simulink model "Fuzzy_and_EKF"  (R2021b)
settings: Solver=ode4  StartTime=0.0  StopTime=25  FixedStep=1e-2  RelTol=1e-3
values from neighbouring files (symbols this model uses):
  n = length(out.tout)    [Plot_dati.m]    (also in sensors_model.m = 2)
undefined symbols (not defined in the file or in its folder): measure
libraries: fuzblock x1
settings Model: Creator=francescoiotti  LastModifiedBy=francescoiotti
settings ModelReferenceCC: ModelReferenceMinAlgLoopOccurrences=on

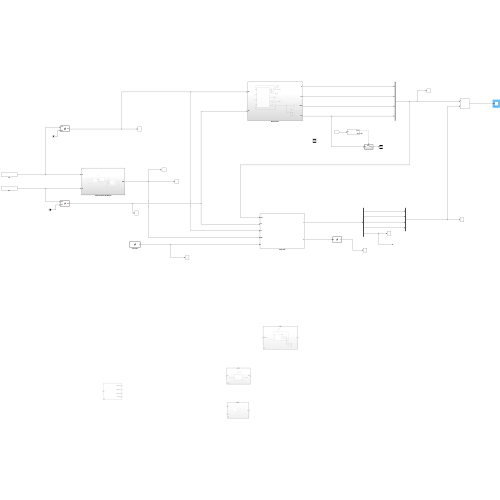
[thumbnail: Simulink's stored preview of the top-level diagram]
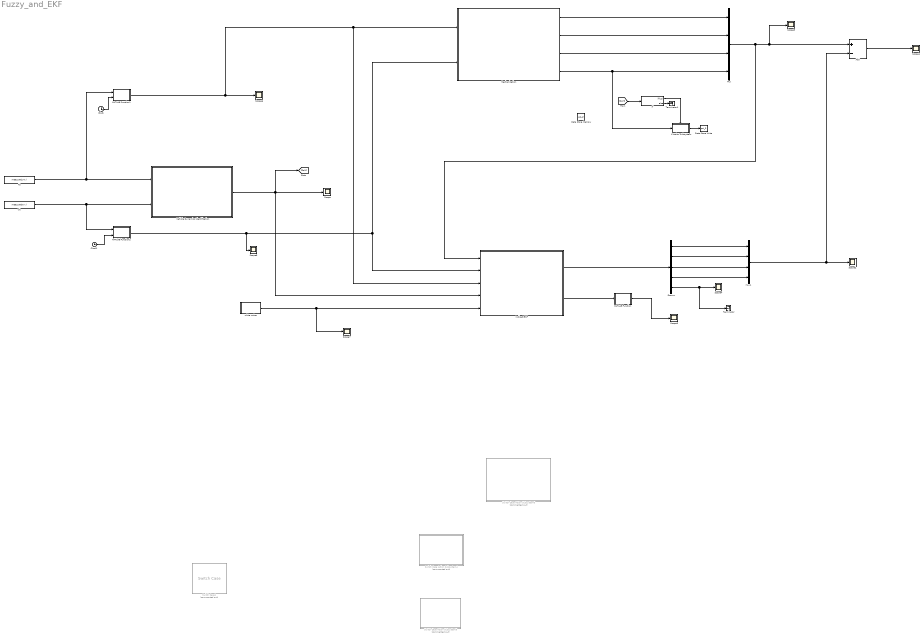
== system Fuzzy_and_EKF ==
  Ab : Constant  Value=measure(2:4,:)
  Add : Sum  Inputs=+-
  Clock : Clock
  Clock1 : Clock
  Data Store Memory : DataStoreMemory  DataStoreName=psi_P  ReadBeforeWriteMsg=warning  WriteAfterWriteMsg=warning  WriteAfterReadMsg=warning  ShowAdditionalParam=off
  Data Store Write : DataStoreWrite  DataStoreName=psi_P  IndexOptions=Index vector (dialog)  Indices=1  OutputSizes=1
  Demux : Demux  Outputs=5
  If : If  IfExpression=u1
  If Action Subsystem : Subsystem  TreatAsAtomicUnit=on
  Indirect EKF : Subsystem
  MATLAB Function : MATLAB Function  TreatAsAtomicUnit=on
  MATLAB Function1 : MATLAB Function  TreatAsAtomicUnit=on
  MATLAB Function2 : MATLAB Function  TreatAsAtomicUnit=on
  Mechanizetion : Subsystem
  Mux : Mux
  Mux1 : Mux
  Scope{,1..8} (9 alike) : Scope
  Switch Case Action Subsystem4 : Subsystem  Commented=on  TreatAsAtomicUnit=on
  Switch Case Action Subsystem5 : Subsystem  Commented=on  TreatAsAtomicUnit=on
  Switch Case Action Subsystem6 : Subsystem  Commented=on  TreatAsAtomicUnit=on
  Switch Case1 : SwitchCase  Commented=on  CaseConditions={0,1,2}
  Terminator : Terminator
  Terminator1 : Terminator
  Vehicle Dynamics Identification : Subsystem
  wb : Constant  Value=measure(5:7,:)
  white noise : MATLAB Function  TreatAsAtomicUnit=on
  wires:
  Vehicle Dynamics Identification/1(SoM) -> Scope/1, [SoM], Indirect EKF/4(SoM)
  Ab/1 -> MATLAB Function1/1(vect), Vehicle Dynamics Identification/1(Ab)
  Indirect EKF/2(P) -> MATLAB Function/1(A)
  white noise/1(u) -> Scope7/1, Indirect EKF/5(u)
  MATLAB Function/1(y) -> Scope3/1
  MATLAB Function1/1(Ab) -> Scope6/1, Indirect EKF/3(Ab), Mechanizetion/1(Ab)
  wb/1 -> MATLAB Function2/1(vect), Vehicle Dynamics Identification/2(wb)
  MATLAB Function2/1(wb) -> Scope8/1, Mechanizetion/2(wb), Indirect EKF/2(wb)
  Clock/1 -> MATLAB Function1/2(time)
  Clock1/1 -> MATLAB Function2/2(time)
  Mux/1 -> Indirect EKF/1(mecc), Scope5/1, Add/1
  Add/1 -> Scope1/1
  Mechanizetion/1(Vf) -> Mux/1
  Mechanizetion/2(phi) -> Mux/2
  Mechanizetion/3(theta) -> Mux/3
  Mechanizetion/4(psi) -> Mux/4, If Action Subsystem/1(psi)
  Indirect EKF/1(x) -> Demux/1
  Demux/1 -> Mux1/1
  Demux/2 -> Mux1/2
  Demux/3 -> Mux1/3
  Demux/4 -> Mux1/4
  Mux1/1 -> Scope2/1, Add/2
  Demux/5 -> Scope4/1, Terminator/1
  [SoM] -> If/1
  If/1 -> If Action Subsystem/Action
  If Action Subsystem/1(psi_P) -> Data Store Write/1
  If/2 -> Terminator1/1

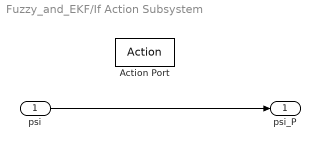
== system Fuzzy_and_EKF/If Action Subsystem ==
  psi : Inport
  Action Port : ActionPort  ActionPortLabel=if(u1)
  psi_P : Outport
  wires:
  psi/1 -> psi_P/1

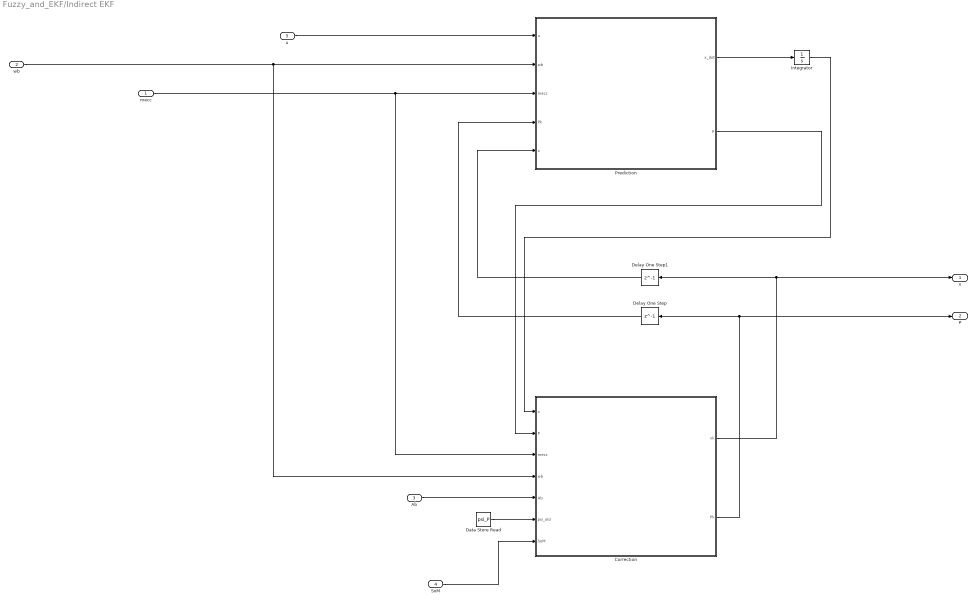
== system Fuzzy_and_EKF/Indirect EKF ==
  mecc : Inport
  wb : Inport  Port=2
  Ab : Inport  Port=3
  SoM : Inport  Port=4
  u : Inport  Port=5
  Correction : MATLAB Function  TreatAsAtomicUnit=on
  Data Store Read : DataStoreRead  DataStoreName=psi_P  IndexOptions=Index vector (dialog)  Indices=1  OutputSizes=1
  Delay One Step : Delay  DelayLength=1
  Delay One Step1 : Delay  DelayLength=1
  Integrator : Integrator  InitialCondition=[0 0 0 0 0]'
  Prediction : MATLAB Function  InitFcn=Pk = eye(5)  TreatAsAtomicUnit=on
  x : Outport
  P : Outport  Port=2
  wires:
  Prediction/1(x_dot) -> Integrator/1
  Integrator/1 -> Correction/1(x)
  SoM/1 -> Correction/7(SoM)
  Correction/1(xk) -> Delay One Step1/1, x/1
  Correction/2(Pk) -> Delay One Step/1, P/1
  Prediction/2(P) -> Correction/2(P)
  Delay One Step/1 -> Prediction/4(Pk)
  Delay One Step1/1 -> Prediction/5(x)
  u/1 -> Prediction/1(u)
  wb/1 -> Correction/4(wb), Prediction/2(wb)
  Ab/1 -> Correction/5(Ab)
  mecc/1 -> Correction/3(mecc), Prediction/3(mecc)
  Data Store Read/1 -> Correction/6(psi_old)

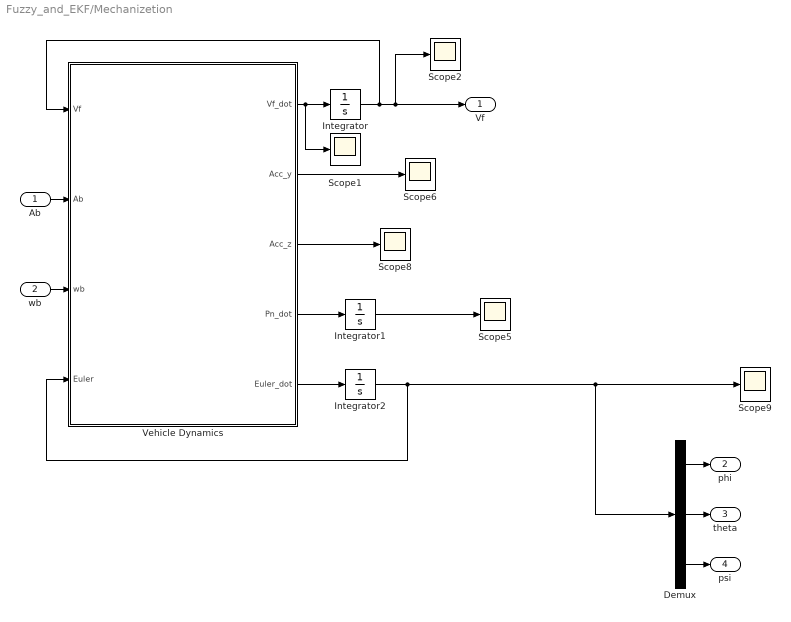
== system Fuzzy_and_EKF/Mechanizetion ==
  Ab : Inport
  wb : Inport  Port=2
  Demux : Demux  Outputs=3
  Integrator : Integrator
  Integrator1 : Integrator  InitialCondition=[0 0 0]'
  Integrator2 : Integrator  InitialCondition=[0 0 0]'
  Scope{1..2,5..6,8..9} (6 alike) : Scope
  Vehicle Dynamics : MATLAB Function  TreatAsAtomicUnit=on
  Vf : Outport
  phi : Outport  Port=2
  theta : Outport  Port=3
  psi : Outport  Port=4
  wires:
  Integrator2/1 -> Vehicle Dynamics/4(Euler), Demux/1, Scope9/1
  Integrator/1 -> Vehicle Dynamics/1(Vf), Vf/1, Scope2/1
  Vehicle Dynamics/3(Acc_z) -> Scope8/1
  Vehicle Dynamics/1(Vf_dot) -> Scope1/1, Integrator/1
  wb/1 -> Vehicle Dynamics/3(wb)
  Vehicle Dynamics/4(Pn_dot) -> Integrator1/1
  Vehicle Dynamics/2(Acc_y) -> Scope6/1
  Integrator1/1 -> Scope5/1
  Vehicle Dynamics/5(Euler_dot) -> Integrator2/1
  Demux/2 -> theta/1
  Demux/3 -> psi/1
  Demux/1 -> phi/1
  Ab/1 -> Vehicle Dynamics/2(Ab)

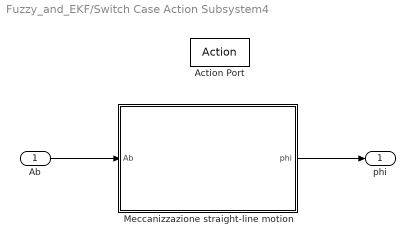
== system Fuzzy_and_EKF/Switch Case Action Subsystem4 ==
  Ab : Inport
  Action Port : ActionPort
  Meccanizzazione straight-line motion : MATLAB Function  TreatAsAtomicUnit=on
  phi : Outport
  wires:
  Ab/1 -> Meccanizzazione straight-line motion/1(Ab)
  Meccanizzazione straight-line motion/1(phi) -> phi/1

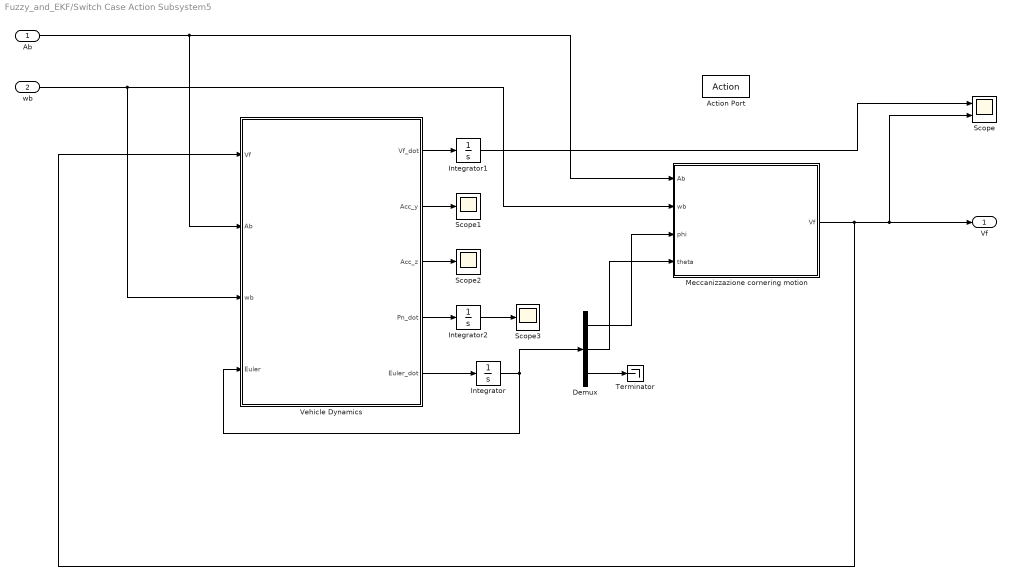
== system Fuzzy_and_EKF/Switch Case Action Subsystem5 ==
  Ab : Inport
  wb : Inport  Port=2
  Action Port : ActionPort
  Demux : Demux  Outputs=3
  Integrator : Integrator  InitialCondition=[0 0 0]'
  Integrator1 : Integrator
  Integrator2 : Integrator  InitialCondition=[0 0 0]'
  Meccanizzazione cornering motion : MATLAB Function  TreatAsAtomicUnit=on
  Scope : Scope  NumInputPorts=2
  Scope1 : Scope
  Scope2 : Scope
  Scope3 : Scope
  Terminator : Terminator
  Vehicle Dynamics : MATLAB Function  TreatAsAtomicUnit=on
  Vf : Outport
  wires:
  Meccanizzazione cornering motion/1(Vf) -> Vehicle Dynamics/1(Vf), Scope/2, Vf/1
  Ab/1 -> Meccanizzazione cornering motion/1(Ab), Vehicle Dynamics/2(Ab)
  wb/1 -> Meccanizzazione cornering motion/2(wb), Vehicle Dynamics/3(wb)
  Vehicle Dynamics/5(Euler_dot) -> Integrator/1
  Integrator/1 -> Demux/1, Vehicle Dynamics/4(Euler)
  Demux/1 -> Meccanizzazione cornering motion/3(phi)
  Demux/2 -> Meccanizzazione cornering motion/4(theta)
  Demux/3 -> Terminator/1
  Vehicle Dynamics/1(Vf_dot) -> Integrator1/1
  Integrator1/1 -> Scope/1
  Vehicle Dynamics/2(Acc_y) -> Scope1/1
  Vehicle Dynamics/3(Acc_z) -> Scope2/1
  Vehicle Dynamics/4(Pn_dot) -> Integrator2/1
  Integrator2/1 -> Scope3/1

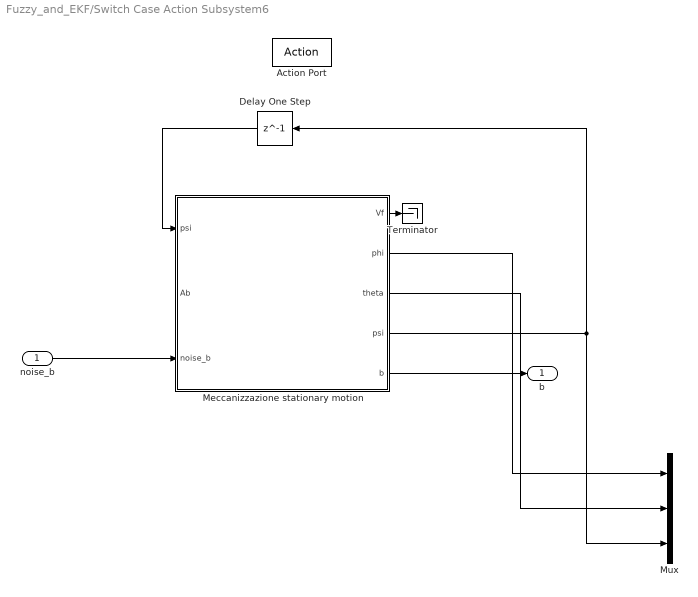
== system Fuzzy_and_EKF/Switch Case Action Subsystem6 ==
  noise_b : Inport
  Action Port : ActionPort
  Delay One Step : Delay  DelayLength=1
  Meccanizzazione stationary motion : MATLAB Function  TreatAsAtomicUnit=on
  Mux : Mux  Inputs=3
  Terminator : Terminator
  b : Outport
  wires:
  noise_b/1 -> Meccanizzazione stationary motion/3(noise_b)
  Meccanizzazione stationary motion/2(phi) -> Mux/1
  Meccanizzazione stationary motion/3(theta) -> Mux/2
  Meccanizzazione stationary motion/4(psi) -> Delay One Step/1, Mux/3
  Meccanizzazione stationary motion/5(b) -> b/1
  Delay One Step/1 -> Meccanizzazione stationary motion/1("psi ")
  Meccanizzazione stationary motion/1(Vf) -> Terminator/1

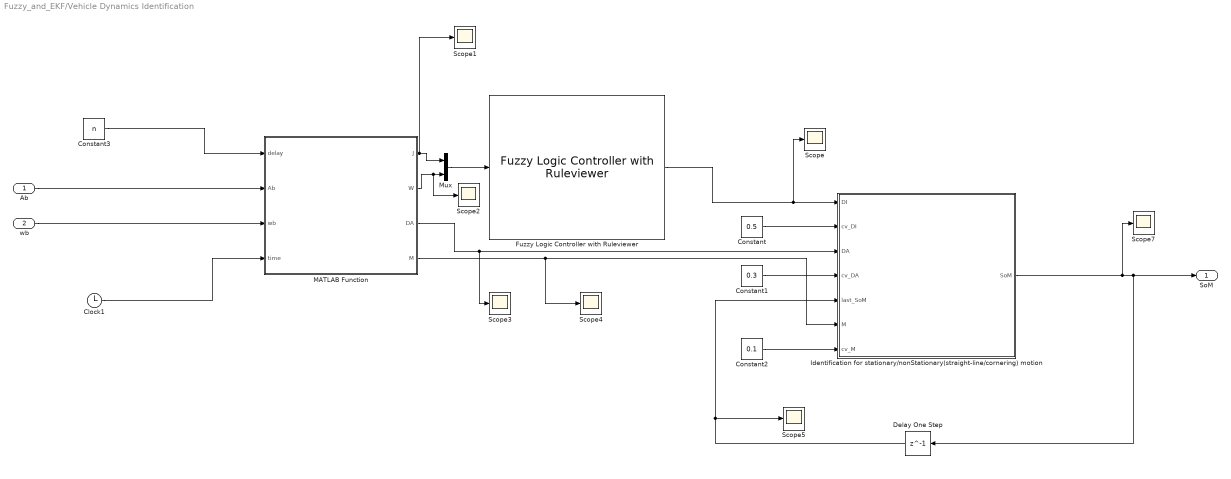
== system Fuzzy_and_EKF/Vehicle Dynamics Identification ==
  Ab : Inport
  wb : Inport  Port=2
  Clock1 : Clock
  Constant : Constant  Value=0.5
  Constant1 : Constant  Value=0.3
  Constant2 : Constant  Value=0.1
  Constant3 : Constant  Value=n
  Delay One Step : Delay  DelayLength=1  InitialCondition=1
  Fuzzy Logic Controller with Ruleviewer : fuzblock/Fuzzy Logic  Controller  with Ruleviewer  fismatrix=pippo  Ts=5
  Identification for stationary/nonStationary(straight-line/cornering) motion : MATLAB Function  TreatAsAtomicUnit=on
  MATLAB Function : MATLAB Function  TreatAsAtomicUnit=on
  Mux : Mux  Inputs=2
  Scope{,1..5,7} (7 alike) : Scope
  SoM : Outport
  wires:
  Constant1/1 -> Identification for stationary/nonStationary(straight-line/cornering) motion/4(cv_DA)
  MATLAB Function/3(DA) -> Scope3/1, Identification for stationary/nonStationary(straight-line/cornering) motion/3(DA)
  MATLAB Function/1(J) -> Scope1/1, Mux/1
  Fuzzy Logic Controller with Ruleviewer/1 -> Scope/1, Identification for stationary/nonStationary(straight-line/cornering) motion/1(DI)
  MATLAB Function/4(M) -> Scope4/1, Identification for stationary/nonStationary(straight-line/cornering) motion/6(M)
  Identification for stationary/nonStationary(straight-line/cornering) motion/1(SoM) -> Scope7/1, SoM/1, Delay One Step/1
  Constant2/1 -> Identification for stationary/nonStationary(straight-line/cornering) motion/7(cv_M)
  Constant/1 -> Identification for stationary/nonStationary(straight-line/cornering) motion/2(cv_DI)
  MATLAB Function/2(W) -> Scope2/1, Mux/2
  Mux/1 -> Fuzzy Logic Controller with Ruleviewer/1
  Clock1/1 -> MATLAB Function/4(time)
  wb/1 -> MATLAB Function/3(wb)
  Ab/1 -> MATLAB Function/2(Ab)
  Constant3/1 -> MATLAB Function/1(delay)
  Delay One Step/1 -> Scope5/1, Identification for stationary/nonStationary(straight-line/cornering) motion/5(last_SoM)

== matlab function Fuzzy_and_EKF/Mechanizetion/Vehicle Dynamics ==
  data: Vf input; Ab input; wb input; Euler input; Vf_dot output; Acc_y output; Acc_z output; Pn_dot output; Euler_dot output
function [Vf_dot, Acc_y, Acc_z, Pn_dot, Euler_dot] = Vehicle_model(Vf, Ab, wb, Euler)
%% Land Vehicle Dynamic model
% x_dot is the derivative of x

Abx = Ab(1);
Aby = Ab(2);
Abz = Ab(3);

wbx = wb(1);
wby = wb(2);
wbz = wb(3);

% Euler angles
phi = Euler(1);
theta = Euler(2);
psi = Euler(3);

% Constant
g = 9.81;

% Model
Vf_dot = Abx - g*sin(theta);
Acc_y = Aby + g*sin(phi)*cos(theta);
Acc_z = -Abz - g*cos(phi)*cos(theta);
phi_dot = wbx + sin(phi)*tan(theta)*wby + cos(phi)*tan(theta)*wbz;
theta_dot = cos(phi)*wby - sin(phi)*wbz;
psi_dot = sin(phi)/cos(theta)*wby + cos(phi)/cos(theta) * wbz;
Pnn_dot = Vf*cos(theta)*cos(psi);
Pne_dot = Vf*cos(theta)*sin(psi);
Pnd_dot = Vf*sin(theta);

Ab = [Abx, Aby, Abz]';
Euler_dot = [phi_dot, theta_dot, psi_dot]';
Pn_dot = [Pnn_dot, Pne_dot, Pnd_dot]';

== matlab function Fuzzy_and_EKF/Switch Case Action Subsystem4/Meccanizzazione straight-line motion ==
  data: Ab input; phi output
function phi  = mecc(Ab)
% Estraggo le componenti di accelerazione
Abx = Ab(1);
Aby = Ab(2);

% Estraggo le componenti di velocità angolare
% wbx = wb(1);
% wby = wb(2);
% wbz = wb(3);

% Costante
g = 9.81;

% Meccanizzazione
phi = asin(-Aby / sqrt(g^2 - Abx^2));

== matlab function Fuzzy_and_EKF/Switch Case Action Subsystem5/Meccanizzazione cornering motion ==
  data: Ab input; wb input; phi input; Vf output; theta input
function Vf  = mecc(Ab, wb, phi, theta)
% Estraggo le componenti di accelerazione
%Abx = Ab(1);
Aby = Ab(2);

% Estraggo le componenti di velocità angolare
% wbx = wb(1);
% wby = wb(2);
wbz = wb(3);

% Costante
g = 9.81;

% Meccanizzazione
Vf = (Aby + g*sin(phi)*cos(theta)) / wbz;

== matlab function Fuzzy_and_EKF/Switch Case Action Subsystem5/Vehicle Dynamics ==
  data: Vf input; Ab input; wb input; Euler input; Vf_dot output; Acc_y output; Acc_z output; Pn_dot output; Euler_dot output
function [Vf_dot, Acc_y, Acc_z, Pn_dot, Euler_dot] = Vehicle_model(Vf, Ab, wb, Euler)
%% Land Vehicle Dynamic model
% x_dot is the derivative of x

Abx = Ab(1);
Aby = Ab(2);
Abz = Ab(3);

wbx = wb(1);
wby = wb(2);
wbz = wb(3);

% Euler angles
phi = Euler(1);
theta = Euler(2);
psi = Euler(3);

% Constant
g = 9.81;

% Model
Vf_dot = Abx - g*sin(theta);
Acc_y = Aby + g*sin(phi)*cos(theta);
Acc_z = -Abz - g*cos(phi)*cos(theta);
phi_dot = wbx + sin(phi)*tan(theta)*wby + cos(phi)*tan(theta)*wbz;
theta_dot = cos(phi)*wby - sin(phi)*wbz;
psi_dot = sin(phi)/cos(theta)*wby + cos(phi)/cos(theta) * wbz;
Pnn_dot = Vf*cos(theta)*cos(psi);
Pne_dot = Vf*cos(theta)*sin(psi);
Pnd_dot = Vf*sin(theta);

Euler_dot = [phi_dot, theta_dot, psi_dot]';
Pn_dot = [Pnn_dot, Pne_dot, Pnd_dot]';

== matlab function Fuzzy_and_EKF/Switch Case Action Subsystem6/Meccanizzazione stationary motion ==
  data: Vf output; phi output; theta output; psi input; psi output; Ab input; noise_b input; b output
function [Vf, phi, theta, psi, b] = mecc(psi, Ab, noise_b)
% Estraggo le componenti di accelerazione
Abx = Ab(1);
Aby = Ab(2);

% Estraggo le componenti di velocità angolare
% wbx = wb(1);
% wby = wb(2);
% wbz = wb(3);

% Costante
g = 9.81;

% Meccanizzazione
theta = asin(Abx/g);
phi = asin(-Aby / sqrt(g^2 - Abx^2));
psi = psi;
Vf = 0;
b = noise_b;

== matlab function Fuzzy_and_EKF/Vehicle Dynamics Identification/Identification for stationary//nonStationary(straight-line//cornering) motion ==
  data: DI input; cv_DI input; DA input; cv_DA input; last_SoM input; M input; SoM output; cv_M input
function SoM = type_of_motion_decision_loop(DI, cv_DI, DA, cv_DA, last_SoM, M, cv_M)

    %% Identification for stationary/nonStationary(straight-line/cornering) motion
    % SoM : state of motion for landend vehicle
    % last_SoM: previous state of motion for landend vehicle
    % 0 := Stationary
    % 1 := straight-line motion
    % 2 := cornering motion
    % notStationary: if 1 the vehicle is not stationary

    notStationary = 1;
    SoM = 0;

    if last_SoM == 0 && DA > cv_DA      
        notStationary = 1;
    elseif	last_SoM && DA < cv_DA && DI < cv_DI
        SoM = 0;
        notStationary = 0;
    else 
        SoM = last_SoM;
        notStationary = 0;
    end
    
    %Run this only if notStactionary
    if notStationary && M > cv_M
        SoM = 2;
    elseif	notStationary && M < cv_M
        SoM = 1;
    elseif notStationary 
        SoM = last_SoM;
    end

== matlab function Fuzzy_and_EKF/Vehicle Dynamics Identification/MATLAB Function ==
  data: delay input; Ab input; J output; wb input; time input; W output; DA output; M output
function [J, W, DA, M] = functional_computation(delay, Ab, wb, time)
% Trasformo i tempi in passi
n = int64(delay/1e-2);
t = int64(time/1e-2);
p = int64(0.2/1e-2);
m = n;
% Inizializzo i funzionali
J = 0;
W = 0;
DA = 0;
Mwbz = 0;

% Calcolo J
for i=t-n:t
%   Controllo nel caso in cui t < n ed escludo i termini con indici
%   negativi
    if i > 1
        J = J + abs( norm(Ab(:,i)) - norm(Ab(:,i-1)) );
    end
end

% Calcolo W
for i=t-n:t
%   Controllo nel caso in cui t < n ed escludo i termini con indici
%   negativi
    if i > 1
        W = W + abs( sqrt(wb(1,i)^2 + wb(2,i)^2) ) / double(n);
    end
end


% Calcolo DA
for i=t-p:t
%   Controllo nel caso in cui t < n ed escludo i termini con indici
%   negativi
    if i > 1 && t-p > 0
        DA = DA + abs( Ab(1,i) - Ab(1,t-p) );
    end
end


% Calcolo M
for i=t-m:t
%   Controllo nel caso in cui t < n ed escludo i termini con indici
%   negativi
    if i > 1
        Mwbz = Mwbz + wb(3,i);
    end
end
M = Mwbz / double(m);

== matlab function Fuzzy_and_EKF/Indirect EKF/Prediction ==
  data: u input; wb input; mecc input; Pk input; x_dot output; x input; P output
function [x_dot, P] = prediction(u, wb, mecc, Pk, x)

% Estraggo le componenti di velocità angolare
wbx = wb(1);
wby = wb(2);
wbz = wb(3);

% Estraggo le grandezze calcolate con la meccanizzazione
Vf = mecc(1);
phi = mecc(2);
theta = mecc(3);
psi = mecc(4);

% Costante
g = 9.81;

% Definisco gli elementi della matrice F
f13 = -g*cos(theta);
f22 = cos(phi)*tan(theta)*wby - sin(phi)*tan(theta)*wbz;
f23 = sin(phi)*wby/cos(theta)^2 + cos(phi)*wbz/cos(theta)^2;
f32 = -sin(phi)*wby - cos(phi)*wbz;
f42 = cos(phi)*wby/cos(theta) - sin(phi)*wbz/cos(theta);
f43 = sin(phi)*tan(theta)*wby/cos(theta) + cos(phi)*tan(theta)*wbz/cos(theta);

F = [0  0  f13  0  1;
     0 f22 f23  0  0;
     0 f32  0   0  0;
     0 f42 f43  0  0;
     0  0   0   0  0;];

% Definisco gli elementi della matrice G
g23 = sin(phi)*tan(theta);
g24 = cos(phi)*tan(theta);
g33 = cos(phi);
g34 = -sin(phi);
g43 = sin(phi)/cos(theta);
g44 = cos(phi)/cos(theta);

G = [1  0  0   0  0;
     0  1 g23 g24 0;
     0  0 g33 g34 0;
     0  0 g43 g44 0;
     0  0  0   0  1;];

% Formula di predizione dello stato
x_dot = F*x + G*u;


% Definisco la matrice di covarianza del rumore di processo Q
qAbx = 0.001; % densità spettrale
qwbx = 0.1;
qwby = 0.1;
qwbz = 0.1;
qb = 0;
Q = diag([qAbx, qwbx, qwby, qwbz, qb]);

% Formula di predizione della covarianza
P = F*Pk*F' + Q;

== matlab function Fuzzy_and_EKF/Indirect EKF/Correction ==
  data: x input; xk output; P input; mecc input; wb input; Ab input; psi_old input; Pk output; SoM input
function [xk, Pk] = correction(x, P, mecc, wb, Ab, psi_old, SoM)
% Estraggo le componenti di accelerazione
Abx = Ab(1);
Aby = Ab(2);
Abz = Ab(3);

% Estraggo le componenti di velocità angolare
wbx = wb(1);
wby = wb(2);
wbz = wb(3);

% Estraggo le grandezze calcolate con la meccanizzazione
Vf = mecc(1);
phi = mecc(2);
theta = mecc(3);
psi = mecc(4);

% Costante
g = 9.81;

% z = [ Vf ; phi-phi_a ; theta-theta_a ; psi-psi_p ]
if SoM == 0

    % Definisco la matrice H
    H = [ 1 0 0 0 0;
          0 1 0 0 0;
          0 0 1 0 0;
          0 0 0 1 0;];
    % Deviazioni standard rumori di misura in fase stazionaria
    sigma_deltaVf_ZUPT = 0.02;
    sigma_deltaPhi = 0.2;
    sigma_deltaTheta = 0.2;
    sigma_deltaPsi = 0.02;
    % Matrice di covarianza
    R = diag([sigma_deltaVf_ZUPT^2, sigma_deltaPhi^2, sigma_deltaTheta^2, sigma_deltaPsi^2]);

    % Misure dynamics-derived
    phi_A = asin(-Aby / sqrt(g^2 - Abx^2));
    theta_A = asin(Abx/g);
    psi_P = psi_old;

    z = [Vf; phi - phi_A; theta - theta_A; psi - psi_P];

elseif SoM == 1

    % Definisco la matrice H
    H = [ 0 1 0 0 0;];

    % Deviazioni standard rumori di misura in fase di movimento lineare
    sigma_deltaPhi = 0.2;
    % Matrice di covarianza
    R = sigma_deltaPhi^2;
    
    % Misure dynamics-derived
    phi_A = asin(-Aby / sqrt(g^2 - Abx^2));

    z = phi - phi_A;

elseif SoM == 2

    % Definisco la matrice H
    H = [ 1 0 0 0 0;];

    % Deviazioni standard rumori di misura in fase di cornering
    sigma_deltaVf_C = 0.02;
    % Matrice di covarianza
    R = sigma_deltaVf_C^2;
    
    % Misure dynamics-derived
    Vf_C = (Aby + g*sin(phi)*cos(theta)) / wbz;

    z = Vf - Vf_C;

else
%   Caso unaided
    H = zeros(4,5);
    R = eye(4);
    z = zeros(4,1);
    fprintf('SoM non si identifica in un genere');

end

% Innovazione
e = z - H * x;
% Covarianza dell'innovazione
S = H * P * H' + R;
L = P * H' * S^(-1);
% Correzione
xk = x + L*e;
% Pk = P - L*S*L';
Pk = (eye(5) - L*H) * P * (eye(5) - L*H)' + L*R*L';

== matlab function Fuzzy_and_EKF/white noise ==
  data: u output
function u = fcn()
% Accelerometer 
stdv_a = 0.0055; % standard deviation
Wna = stdv_a*randn(1,1); % White Noise
% Gyroscope
stdv_g = 0.6325; % standard deviation
Wng = stdv_g*randn(1,3); % White Noise

u = [Wna, Wng, 0]';

== matlab function Fuzzy_and_EKF/MATLAB Function ==
  data: A input; y output
function y = fcn(A)
y = norm(A);

== matlab function Fuzzy_and_EKF/MATLAB Function1 ==
  data: vect input; Ab output; time input
function Ab = fcn(vect, time)
t = int64(time/1e-2)+1;
Ab = vect(:,t);

== matlab function Fuzzy_and_EKF/MATLAB Function2 ==
  data: vect input; time input; wb output
function wb = fcn(vect, time)
t = int64(time/1e-2)+1;
wb = vect(:,t);
